simulink model "insulin_model"  (R2022a)
settings: Solver=VariableStepAuto  StartTime=0.0  StopTime=10.0  RelTol=1e-3
undefined symbols (not defined in the file): G, Gb, I, Ib, k3, k4, tau
settings Model: Creator=dell  LastModifiedBy=dell

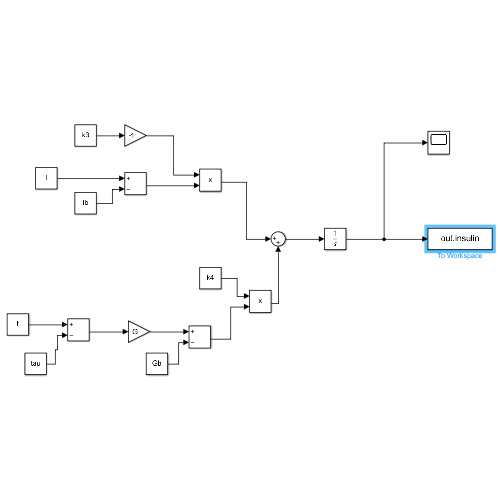
[thumbnail: Simulink's stored preview of the top-level diagram]
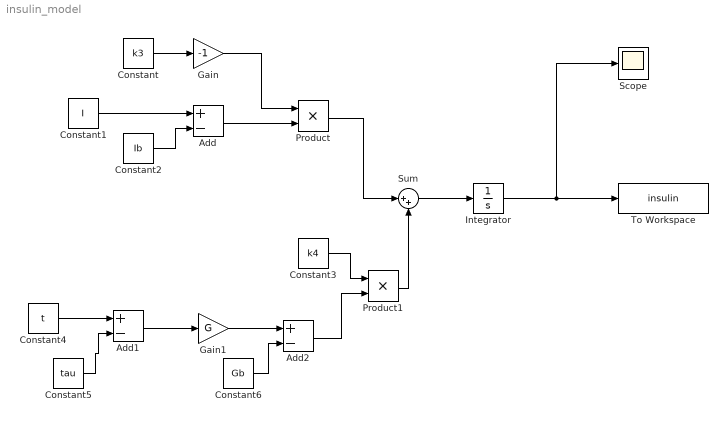
== system insulin_model ==
  Add : Sum  Inputs=+-
  Add1 : Sum  Inputs=+-
  Add2 : Sum  Inputs=+-
  Constant : Constant  Value=k3
  Constant1 : Constant  Value=I
  Constant2 : Constant  Value=Ib
  Constant3 : Constant  Value=k4
  Constant4 : Constant  Value=t
  Constant5 : Constant  Value=tau
  Constant6 : Constant  Value=Gb
  Gain : Gain  Gain=-1
  Gain1 : Gain  Gain=G
  Integrator : Integrator
  Product : Product
  Product1 : Product
  Scope : Scope
  Sum : Sum  Inputs=|++
  To Workspace : ToWorkspace  VariableName=insulin  SaveFormat=Timeseries  SampleTime=-1
  wires:
  Product/1 -> Sum/1
  Constant2/1 -> Add/2
  Constant1/1 -> Add/1
  Constant/1 -> Gain/1
  Gain/1 -> Product/1
  Add/1 -> Product/2
  Product1/1 -> Sum/2
  Constant4/1 -> Add1/1
  Constant5/1 -> Add1/2
  Constant3/1 -> Product1/1
  Add1/1 -> Gain1/1
  Gain1/1 -> Add2/1
  Constant6/1 -> Add2/2
  Add2/1 -> Product1/2
  Sum/1 -> Integrator/1
  Integrator/1 -> To Workspace/1, Scope/1
